simulink model "GScaleModelTrain_FuelCell"  (R2025b)
settings: Solver=ode23t  StartTime=0.0  StopTime=10  FixedStep=0.001  RelTol=1e-3
values from neighbouring files (symbols this model uses):
  eff = 0.85    [GScaleModelMatlab.m]
  G = 30    [GScaleModelMatlab.m]
  Ke = 0.01275    [GScaleModelMatlab.m]
  Kt = 0.01275    [GScaleModelMatlab.m]
  L = 0.001    [GScaleModelMatlab.m]
  num_motors = 2    [GScaleModelMatlab.m]
  num_wheels = 8    [GScaleModelMatlab.m]
  r = 0.017    [GScaleModelMatlab.m]
  Rm = 2.1    [GScaleModelMatlab.m]
  train_mass = mass_loco + (N * mass_wag)    (= 10.5)    [DavisResistance.m]    (also in GScaleModelMatlab.m)
  Vtrack = 20    [GScaleModelMatlab.m]
  x01 = 0    [GScaleModelMatlab.m]
  x02 = -0.5225    [GScaleModelMatlab.m]
  x03 = -1.1225    [GScaleModelMatlab.m]
  x04 = -1.7225    [GScaleModelMatlab.m]
libraries: fl_lib x12, nesl_utility x11, ee_lib x4
settings Model: Creator=2311591M  LastModifiedBy=Rahul
settings DebuggingCC: AlgebraicLoopMsg=none
settings SimscapeCC: SimscapeLogType=all

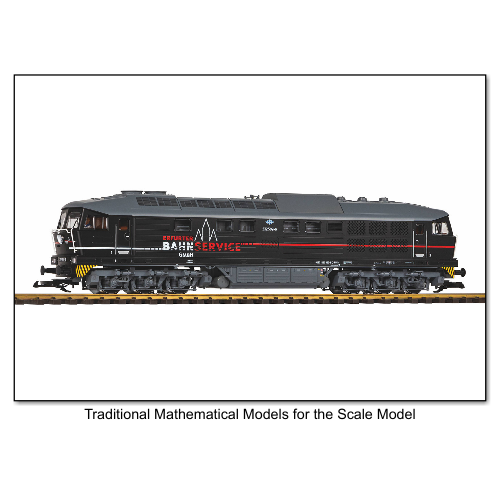
[thumbnail: Simulink's stored preview of the top-level diagram]
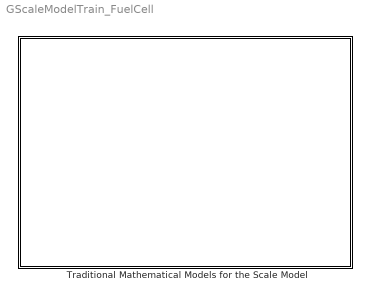
== system GScaleModelTrain_FuelCell ==
  Traditional Mathematical Models for the Scale Model : Subsystem
      mask Display: image('Luddy.jpg');

== system GScaleModelTrain_FuelCell/Traditional Mathematical Models for the Scale Model ==
  Combined Mass System : Subsystem
  Distributed Mass System : Subsystem
  Speed Visual : Scope  NumInputPorts=2
      settings: ActiveDisplayYMinimum=0.078796061919818139  ActiveDisplayYMaximum=1.1196711774107109  YLabel=Speed (m/s)  DataLoggingVariableName=ScopeData_3
  wires:
  Distributed Mass System/1(xd1) -> Speed Visual/2  "Distributed"
  Combined Mass System/1(xd) -> Speed Visual/1  "Combined"

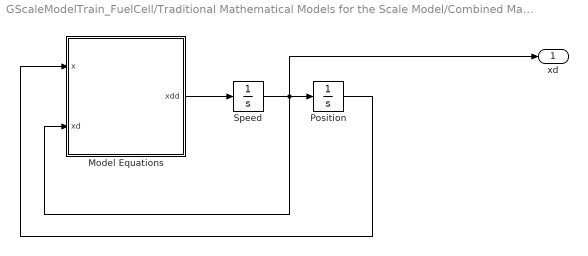
== system GScaleModelTrain_FuelCell/Traditional Mathematical Models for the Scale Model/Combined Mass System ==
  Model Equations : Subsystem
  Position : Integrator
  Speed : Integrator
  xd : Outport
  wires:
  Position/1 -> Model Equations/1(x)
  Model Equations/1(xdd) -> Speed/1
  Speed/1 -> xd/1, Model Equations/2(xd), Position/1

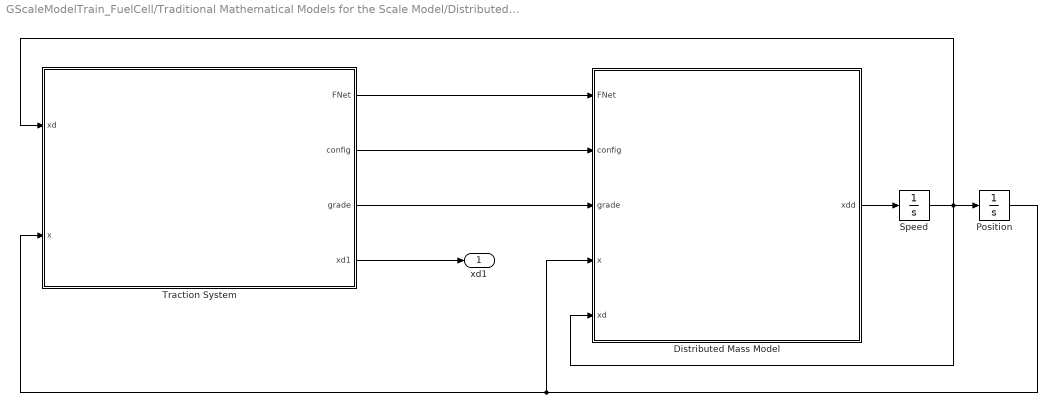
== system GScaleModelTrain_FuelCell/Traditional Mathematical Models for the Scale Model/Distributed Mass System ==
  Distributed Mass Model : MATLAB Function  TreatAsAtomicUnit=on
  Position : Integrator  InitialCondition=[x01; x02; x03; x04]
  Speed : Integrator
  Traction System : Subsystem
  xd1 : Outport
  wires:
  Traction System/4(xd1) -> xd1/1
  Traction System/3(grade) -> Distributed Mass Model/3(grade)
  Traction System/2(config) -> Distributed Mass Model/2(config)
  Traction System/1(FNet) -> Distributed Mass Model/1(FNet)
  Position/1 -> Distributed Mass Model/4(x), Traction System/2(x)
  Speed/1 -> Traction System/1(xd), Distributed Mass Model/5(xd), Position/1
  Distributed Mass Model/1(xdd) -> Speed/1

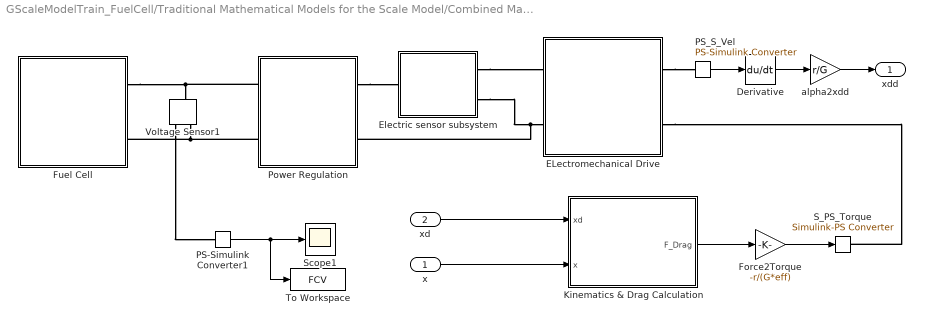
== system GScaleModelTrain_FuelCell/Traditional Mathematical Models for the Scale Model/Combined Mass System/Model Equations ==
  x : Inport
  xd : Inport  Port=2
  Derivative : Derivative
  ELectromechanical Drive : Subsystem
  Electric sensor subsystem : Subsystem
  Force2Torque : Gain  Gain=-r/(G*eff)
  Fuel Cell : Subsystem
  Kinematics & Drag Calculation : Subsystem
  PS-Simulink Converter1 : nesl_utility/PS-Simulink Converter  PhysicalDomain=network_engine_domain  SubClassName=ps_output  LeftPortType=input  RightPortType=output  PseudoPeriodic=off  Frequencies=[]  VectorFormat=inherit  Unit=inherit  AffineConversion=off
  PS_S_Vel : nesl_utility/PS-Simulink Converter  PhysicalDomain=network_engine_domain  SubClassName=ps_output  LeftPortType=input  RightPortType=output  PseudoPeriodic=off  Frequencies=[]  VectorFormat=inherit  Unit=inherit  AffineConversion=off
  Power Regulation : Subsystem
  S_PS_Torque : nesl_utility/Simulink-PS Converter  PhysicalDomain=network_engine_domain  SubClassName=ps_input  LeftPortType=input  RightPortType=output  PseudoPeriodic=off  Frequencies=[]  NoiseDistribution=none  NoiseParameters=[]  Unit=1  AffineConversion=off  FilteringAndDerivatives=filter  SimscapeFilterOrder=1  InputFilterTimeConstant=0.001  UdotUserProvided=0
  Scope1 : Scope
      settings: ActiveDisplayYMinimum=14.64179812710913  ActiveDisplayYMaximum=19.590394326626626
  To Workspace : ToWorkspace  VariableName=FCV  SaveFormat=Timeseries  SampleTime=-1
  Voltage Sensor1 : fl_lib/Electrical/Electrical Sensors/Voltage Sensor
  alpha2xdd : Gain  Gain=r/G
  xdd : Outport
  wires:
  Force2Torque/1 -> S_PS_Torque/1
  Derivative/1 -> alpha2xdd/1
  alpha2xdd/1 -> xdd/1
  PS_S_Vel/1 -> Derivative/1
  PS-Simulink Converter1/1 -> To Workspace/1, Scope1/1
  x/1 -> Kinematics & Drag Calculation/2(x)
  xd/1 -> Kinematics & Drag Calculation/1(xd)
  Kinematics & Drag Calculation/1(F_Drag) -> Force2Torque/1
  connections:
  Fuel Cell/RConn1 -- Power Regulation/LConn1 -- Voltage Sensor1/LConn1
  Voltage Sensor1/RConn1 -- PS-Simulink Converter1/LConn1
  Voltage Sensor1/RConn2 -- Fuel Cell/RConn2 -- Power Regulation/LConn2
  ELectromechanical Drive/RConn1 -- PS_S_Vel/LConn1
  ELectromechanical Drive/RConn2 -- S_PS_Torque/RConn1
  ELectromechanical Drive/LConn2 -- Electric sensor subsystem/RConn2 -- Power Regulation/RConn2
  Power Regulation/RConn1 -- Electric sensor subsystem/LConn1
  Electric sensor subsystem/RConn1 -- ELectromechanical Drive/LConn1

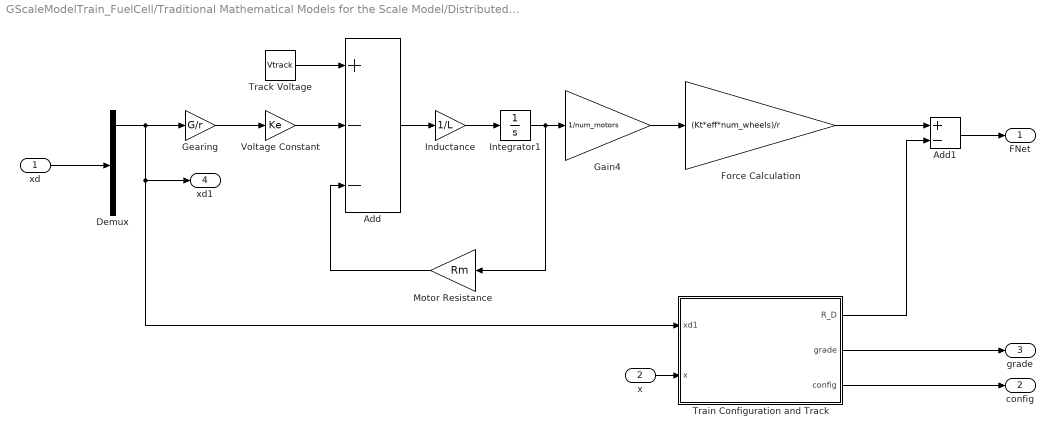
== system GScaleModelTrain_FuelCell/Traditional Mathematical Models for the Scale Model/Distributed Mass System/Traction System ==
  xd : Inport
  x : Inport  Port=2
  Add : Sum  Inputs=+--
  Add1 : Sum  Inputs=+-
  Demux : Demux
  Force Calculation : Gain  Gain=(Kt*eff*num_wheels)/r
  Gain4 : Gain  Gain=1/num_motors
  Gearing : Gain  Gain=G/r
  Inductance : Gain  Gain=1/L
  Integrator1 : Integrator
  Motor Resistance : Gain  Gain=Rm
  Track Voltage : Constant  Value=Vtrack
  Train Configuration and Track : Subsystem
  Voltage Constant : Gain  Gain=Ke
  FNet : Outport
  config : Outport  Port=2
  grade : Outport  Port=3
  xd1 : Outport  Port=4
  wires:
  Motor Resistance/1 -> Add/3
  Demux/1 -> Train Configuration and Track/1(xd1), xd1/1, Gearing/1
  Add/1 -> Inductance/1
  Inductance/1 -> Integrator1/1
  Voltage Constant/1 -> Add/2
  Gain4/1 -> Force Calculation/1
  Integrator1/1 -> Gain4/1, Motor Resistance/1
  Gearing/1 -> Voltage Constant/1
  Force Calculation/1 -> Add1/1
  xd/1 -> Demux/1
  Add1/1 -> FNet/1
  Track Voltage/1 -> Add/1
  x/1 -> Train Configuration and Track/2(x)
  Train Configuration and Track/1(R_D) -> Add1/2
  Train Configuration and Track/2(grade) -> grade/1
  Train Configuration and Track/3(config) -> config/1

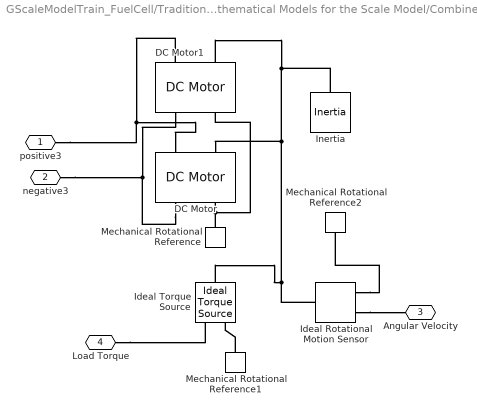
== system GScaleModelTrain_FuelCell/Traditional Mathematical Models for the Scale Model/Combined Mass System/Model Equations/ELectromechanical Drive ==
  DC Motor : ee_lib/Electromechanical/Brushed Motors/DC Motor  field_option=ee.enum.field_option.pm  Rf=100 Ohm  Lf=1 H  Laf=0.15 H  If0=0 A  parameterization=ee.enum.dcparam_option.circuit_param  Ra=Rm Ohm  La=L H  emf_or_torque=ee.enum.emf_or_torque.kv  Kv=Ke V/(rad/s)  Ki=0.01275 N*m/A  T_stall=0.24e-3 N*m  w_max=19100 rpm  w_rated=15000 rpm  P_rated=0.08 W  V_rated=1.5 V  lam_param=ee.enum.lam_param.damping  i_noload=0 A  V_i_noload=1.5 V  J=0.01 cm^2*g  lam=0 N*m*s/rad  speed0=0 rpm  alpha=3.93e-3 1/K  Tmeas=25 degC  thermal_mass=100 J/K  initial_temperature=25 degC
  DC Motor1 : ee_lib/Electromechanical/Brushed Motors/DC Motor  field_option=ee.enum.field_option.pm  Rf=100 Ohm  Lf=1 H  Laf=0.15 H  If0=0 A  parameterization=ee.enum.dcparam_option.circuit_param  Ra=Rm Ohm  La=L H  emf_or_torque=ee.enum.emf_or_torque.kv  Kv=Ke V/(rad/s)  Ki=0.01275 N*m/A  T_stall=0.24e-3 N*m  w_max=19100 rpm  w_rated=15000 rpm  P_rated=0.08 W  V_rated=1.5 V  lam_param=ee.enum.lam_param.damping  i_noload=0 A  V_i_noload=1.5 V  J=0.01 cm^2*g  lam=0 N*m*s/rad  speed0=0 rpm  alpha=3.93e-3 1/K  Tmeas=25 degC  thermal_mass=100 J/K  initial_temperature=25 degC
  Ideal Rotational Motion Sensor : fl_lib/Mechanical/Mechanical Sensors/Ideal Rotational Motion Sensor  reference=foundation.enum.MeasurementReference.difference  acceleration_port=false  velocity_port=true  position_port=false  wrap_angle=false  offset=0 rad
      settings: InternalSimscapePortConfiguration="{\"Bottom\":[],\"Left\":[{\"id\":\"R\",\"label\":\"R\",\"type\":\"foundation.mechanical.rotational.rotational\"}],\"Right\":[{\"id\":\"C\",\"label\":\"C\",\"type\":\"foundation.mechanical.rotational.rotational\"},{\"id\":\"W\",\"label\":\"W\",\"type\":\"output\"}],\"Top\":[]}"
  Ideal Torque Source : fl_lib/Mechanical/Mechanical Sources/Ideal Torque Source
  "Inertia " : fl_lib/Mechanical/Rotational Elements/Inertia  inertia=(train_mass * ( (r/G)^2) ) kg*m^2  num_ports=foundation.enum.numPorts2.one  w_specify=off  w_priority=High  w=0 rad/s  w_nominal_specify=off  w_nominal_value=1  w_nominal_unit=rad/s  t_specify=off  t_priority=None  t=0 N*m  t_nominal_specify=off  t_nominal_value=1  t_nominal_unit=N*m
  Mechanical Rotational Reference : fl_lib/Mechanical/Rotational Elements/Mechanical Rotational Reference
  Mechanical Rotational Reference1 : fl_lib/Mechanical/Rotational Elements/Mechanical Rotational Reference
  Mechanical Rotational Reference2 : fl_lib/Mechanical/Rotational Elements/Mechanical Rotational Reference
  positive3 : PMIOPort  Side=Left
  negative3 : PMIOPort  Port=2  Side=Left
  Angular Velocity : PMIOPort  Port=3  Side=Right
  Load Torque : PMIOPort  Port=4  Side=Right
  connections:
  DC Motor/RConn1 -- negative3/RConn1 -- DC Motor1/RConn1
  Mechanical Rotational Reference/LConn1 -- DC Motor1/RConn2 -- DC Motor/RConn2
  DC Motor1/LConn2 -- Ideal Torque Source/LConn1 -- Ideal Rotational Motion Sensor/LConn1 -- DC Motor/LConn2 -- "Inertia "/LConn1
  Ideal Rotational Motion Sensor/RConn2 -- Angular Velocity/RConn1
  Ideal Rotational Motion Sensor/RConn1 -- Mechanical Rotational Reference2/LConn1
  DC Motor1/LConn1 -- positive3/RConn1 -- DC Motor/LConn1
  Load Torque/RConn1 -- Ideal Torque Source/RConn1
  Mechanical Rotational Reference1/LConn1 -- Ideal Torque Source/RConn2

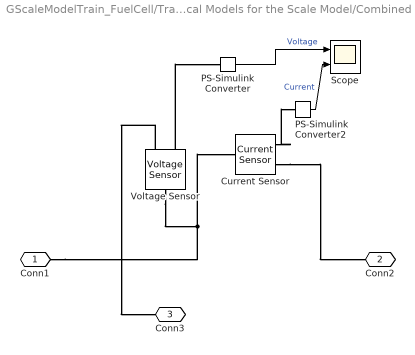
== system GScaleModelTrain_FuelCell/Traditional Mathematical Models for the Scale Model/Combined Mass System/Model Equations/Electric sensor subsystem ==
  Current Sensor : fl_lib/Electrical/Electrical Sensors/Current Sensor
  PS-Simulink Converter : nesl_utility/PS-Simulink Converter  PhysicalDomain=network_engine_domain  SubClassName=ps_output  LeftPortType=input  RightPortType=output  PseudoPeriodic=off  Frequencies=[]  VectorFormat=inherit  Unit=inherit  AffineConversion=off
  PS-Simulink Converter2 : nesl_utility/PS-Simulink Converter  PhysicalDomain=network_engine_domain  SubClassName=ps_output  LeftPortType=input  RightPortType=output  PseudoPeriodic=off  Frequencies=[]  VectorFormat=inherit  Unit=inherit  AffineConversion=off
  Scope : Scope  NumInputPorts=2
      settings: ActiveDisplayYMinimum=-1.7500040602157951  ActiveDisplayYMaximum=15.75003654394216  DataLoggingVariableName=ScopeData_1
  Voltage Sensor : fl_lib/Electrical/Electrical Sensors/Voltage Sensor
  Conn1 : PMIOPort  Side=Left
  Conn2 : PMIOPort  Port=2  Side=Right
  Conn3 : PMIOPort  Port=3  Side=Right
  wires:
  PS-Simulink Converter2/1 -> Scope/2  "Current"
  PS-Simulink Converter/1 -> Scope/1  "Voltage"
  connections:
  Current Sensor/RConn1 -- PS-Simulink Converter2/LConn1
  Voltage Sensor/RConn2 -- Conn3/RConn1
  Voltage Sensor/LConn1 -- Conn1/RConn1 -- Current Sensor/LConn1
  Voltage Sensor/RConn1 -- PS-Simulink Converter/LConn1
  Current Sensor/RConn2 -- Conn2/RConn1

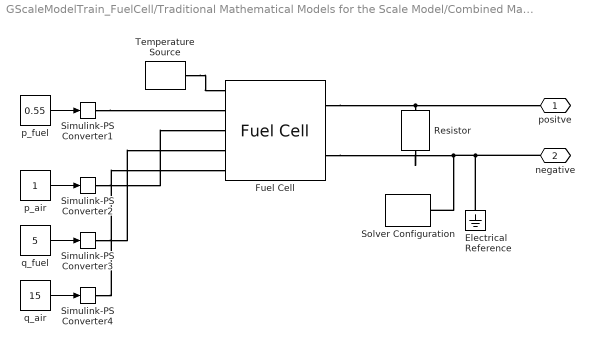
== system GScaleModelTrain_FuelCell/Traditional Mathematical Models for the Scale Model/Combined Mass System/Model Equations/Fuel Cell ==
  Electrical Reference : fl_lib/Electrical/Electrical Elements/Electrical Reference
  Fuel Cell : ee_lib/Sources/Fuel Cell  model_fidelity=ee.enum.fuelcell.fidelity.detailed  Eoc=19.1 V  A=0.125 V  ri=0.2 Ohm  i0=0.1 A  i_lim=10 A  N_cell=20  number_unit=1  pH2_nom=0.55 bar  pO2_nom=1 bar  xH2=99  xO2=21  xW=1  dyn=ee.enum.include.no  Rd=0.005 Ohm  tau=10 s  Tnom=293.15 K  thermal_mass=30000 J/K  iFC_specify=off  iFC_priority=None  iFC=1 A  iFC_nominal_specify=off  iFC_nominal_value=1  iFC_nominal_unit=A  vFC_specify=off  vFC_priority=None  vFC=0 V  vFC_nominal_specify=off  vFC_nominal_value=1  vFC_nominal_unit=V  temperature_specify=off  temperature_priority=High  temperature=293 K  temperature_nominal_specify=off  temperature_nominal_value=1  temperature_nominal_unit=K
      settings: InternalSimscapePortConfiguration="{\"Bottom\":[],\"Left\":[{\"id\":\"H\",\"label\":\"H\",\"type\":\"foundation.thermal.thermal\"},{\"id\":\"pfuel\",\"label\":\"pfuel\",\"type\":\"input\"},{\"id\":\"pair\",\"label\":\"pair\",\"type\":\"input\"},{\"id\":\"qfuel\",\"label\":\"qfuel\",\"type\":\"input\"},{\"id\":\"qair\",\"label\":\"qair\",\"type\":\"input\"}],\"Right\":[{\"id\":\"p\",\"label\":\"+\",\"type\":\"foundation.electrical.electrical\"},{\"id\":\"n\",\"label\":\"-\",\"type\":\"foundation.electrical.electrical\"}],\"Top\":[]}"
  Resistor : fl_lib/Electrical/Electrical Elements/Resistor  R=1000 Ohm  i_specify=off  i_priority=None  i=0 A  i_nominal_specify=off  i_nominal_value=1  i_nominal_unit=A  v_specify=off  v_priority=None  v=0 V  v_nominal_specify=off  v_nominal_value=1  v_nominal_unit=V
  Simulink-PS Converter1 : nesl_utility/Simulink-PS Converter  PhysicalDomain=network_engine_domain  SubClassName=ps_input  LeftPortType=input  RightPortType=output  PseudoPeriodic=off  Frequencies=[]  NoiseDistribution=none  NoiseParameters=[]  Unit=bar  AffineConversion=off  FilteringAndDerivatives=provide  SimscapeFilterOrder=1  InputFilterTimeConstant=0.001  UdotUserProvided=0
  Simulink-PS Converter2 : nesl_utility/Simulink-PS Converter  PhysicalDomain=network_engine_domain  SubClassName=ps_input  LeftPortType=input  RightPortType=output  PseudoPeriodic=off  Frequencies=[]  NoiseDistribution=none  NoiseParameters=[]  Unit=bar  AffineConversion=off  FilteringAndDerivatives=provide  SimscapeFilterOrder=1  InputFilterTimeConstant=0.001  UdotUserProvided=0
  Simulink-PS Converter3 : nesl_utility/Simulink-PS Converter  PhysicalDomain=network_engine_domain  SubClassName=ps_input  LeftPortType=input  RightPortType=output  PseudoPeriodic=off  Frequencies=[]  NoiseDistribution=none  NoiseParameters=[]  Unit=lpm  AffineConversion=off  FilteringAndDerivatives=provide  SimscapeFilterOrder=1  InputFilterTimeConstant=0.001  UdotUserProvided=0
  Simulink-PS Converter4 : nesl_utility/Simulink-PS Converter  PhysicalDomain=network_engine_domain  SubClassName=ps_input  LeftPortType=input  RightPortType=output  PseudoPeriodic=off  Frequencies=[]  NoiseDistribution=none  NoiseParameters=[]  Unit=lpm  AffineConversion=off  FilteringAndDerivatives=provide  SimscapeFilterOrder=1  InputFilterTimeConstant=0.001  UdotUserProvided=0
  Solver Configuration : nesl_utility/Solver Configuration  PhysicalDomain=network_engine_domain  SubClassName=solver  LeftPortType=input  RightPortType=generic  Tones=[]  Harmonics=[]  SimulateNoise=off  Profile=off  UseLocalSampling=off  EnableSwitchedLinearOptims=on  FrequencyDomain=off  UseCCode=off  RelTol=0.001  AbsTol=0.001  MinStep=1e-09  ToWorkspace=off  RevertToSquareIcSolve=off  NumHomotopyIterations=100  PhasorMode=off  PhasorModeNumHarmonics=1  ConsistencySolver=NEWTON_XTOL_AFTER_FTOL  IndexReductionMethod=DerivativeReplacement  DoDC=off  ResidualTolerance=1e-09  ConsistencyTolSource=GLOBAL  ConsistencyAbsTol=0.001  ConsistencyRelTol=0.001  ConsistencyTolFactor=0.001  UseLocalSolver=off  LocalSolverChoice=NE_BACKWARD_EULER_ADVANCER  ResolveIndetEquations=on  FunctionEvalNumThread=1  LocalSolverSampleTime=0.001  DoFixedCost=off  MaxNonlinIter=3  MaxModeIter=2  ComputeImpulses=off  ImpulseIterations=2  LinearAlgebra=auto  LinearAlgebraNumThread=0  EquationFormulation=NE_TIME_EF  DelaysMemoryBudget=1024  AutomaticFiltering=on  FilteringTimeConstant=0.001  PartitionStorageMethod=AS_NEEDED  PartitionMemoryBudget=1024  PartitionMethod=ROBUST  MultibodyUseLocalSolver=off  MultibodyLocalSolverChoice=ODE1  MultibodyLocalSolverSampleTime=0.001
  Temperature Source : fl_lib/Thermal/Thermal Sources/Temperature Source  temperature=293.15 K
  p_air : Constant
  p_fuel : Constant  Value=0.55
  q_air : Constant  Value=15
  q_fuel : Constant  Value=5
  positve : PMIOPort  Side=Right
  negative : PMIOPort  Port=2  Side=Right
  wires:
  p_fuel/1 -> Simulink-PS Converter1/1
  q_air/1 -> Simulink-PS Converter4/1
  q_fuel/1 -> Simulink-PS Converter3/1
  p_air/1 -> Simulink-PS Converter2/1
  connections:
  Electrical Reference/LConn1 -- negative/RConn1 -- Solver Configuration/RConn1 -- Resistor/RConn1 -- Fuel Cell/RConn2
  Temperature Source/LConn1 -- Fuel Cell/LConn1
  Simulink-PS Converter1/RConn1 -- Fuel Cell/LConn2
  Fuel Cell/RConn1 -- Resistor/LConn1 -- positve/RConn1
  Simulink-PS Converter4/RConn1 -- Fuel Cell/LConn5
  Simulink-PS Converter2/RConn1 -- Fuel Cell/LConn3
  Simulink-PS Converter3/RConn1 -- Fuel Cell/LConn4

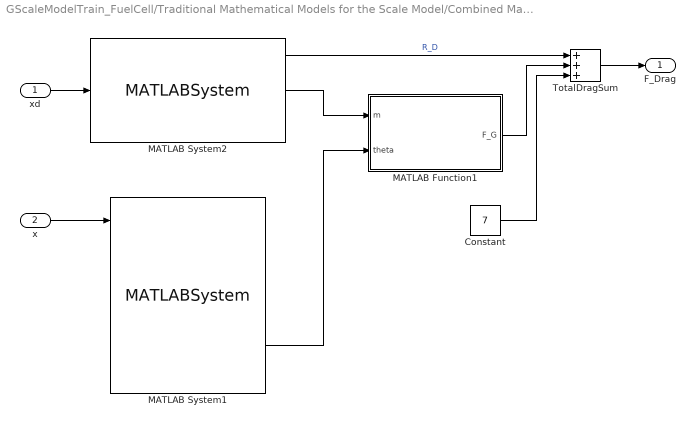
== system GScaleModelTrain_FuelCell/Traditional Mathematical Models for the Scale Model/Combined Mass System/Model Equations/Kinematics & Drag Calculation ==
  xd : Inport
  x : Inport  Port=2
  Constant : Constant  Value=7
  MATLAB Function1 : MATLAB Function  TreatAsAtomicUnit=on
  MATLAB System1 : MATLABSystem  System=Track  SimulateUsing=Code generation
      mask Type: Track
  MATLAB System2 : MATLABSystem  System=DavisResistance  SimulateUsing=Code generation
      mask Type: DavisResistance
  TotalDragSum : Sum  Inputs=+++
  F_Drag : Outport
  wires:
  MATLAB System2/2 -> MATLAB Function1/1(m)
  x/1 -> MATLAB System1/1
  MATLAB System1/2 -> MATLAB Function1/2(theta)
  xd/1 -> MATLAB System2/1
  Constant/1 -> TotalDragSum/3
  MATLAB Function1/1(F_G) -> TotalDragSum/2
  TotalDragSum/1 -> F_Drag/1
  MATLAB System2/1 -> TotalDragSum/1  "R_D"

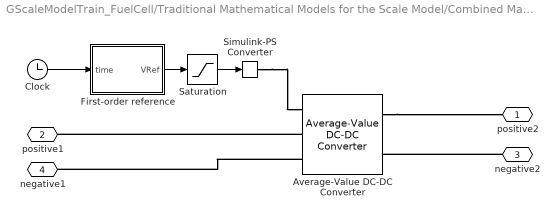
== system GScaleModelTrain_FuelCell/Traditional Mathematical Models for the Scale Model/Combined Mass System/Model Equations/Power Regulation ==
  Average-Value DC-DC Converter : ee_lib/Semiconductors & Converters/Converters/Average-Value DC-DC Converter  implementation_option=ee.enum.converters.implementation.behavioral  converter_type=ee.enum.converters.dcdctype.buck  control_option=ee.enum.converters.controlinput.voltage  efficiency_option=ee.enum.converters.efficiency.constant  efficiency_fixed=100  i_vec=[0, 2, 5] A  efficiency_vec=[90, 95, 98]  Lf=1e-6 H  Rl=1e-3 Ohm  Cf=1e-7 F  Rc=1e-3 Ohm  iL_specify=off  iL_priority=High  iL=0 A  iL_nominal_specify=off  iL_nominal_value=1  iL_nominal_unit=A  vc_specify=on  vc_priority=High  vc=0 V  vc_nominal_specify=on  vc_nominal_value=0  vc_nominal_unit=V
      settings: InternalSimscapePortConfiguration="{\"Bottom\":[],\"Left\":[{\"id\":\"Vref\",\"label\":\"Vref\",\"type\":\"input\"},{\"id\":\"p1\",\"label\":\"1+\",\"type\":\"foundation.electrical.electrical\"},{\"id\":\"n1\",\"label\":\"1-\",\"type\":\"foundation.electrical.electrical\"}],\"Right\":[{\"id\":\"p2\",\"label\":\"2+\",\"type\":\"foundation.electrical.electrical\"},{\"id\":\"n2\",\"label\":\"2-\",\"type\":\"foundation.electrical.electrical\"}],\"Top\":[]}"
  Clock : Clock
  First-order reference : MATLAB Function  TreatAsAtomicUnit=on
  Saturation : Saturate  UpperLimit=14  LowerLimit=0.1
  Simulink-PS Converter : nesl_utility/Simulink-PS Converter  PhysicalDomain=network_engine_domain  SubClassName=ps_input  LeftPortType=input  RightPortType=output  PseudoPeriodic=off  Frequencies=[]  NoiseDistribution=none  NoiseParameters=[]  Unit=V  AffineConversion=off  FilteringAndDerivatives=filter  SimscapeFilterOrder=1  InputFilterTimeConstant=0.001  UdotUserProvided=0
  positive2 : PMIOPort  Side=Right
  positive1 : PMIOPort  Port=2  Side=Left
  negative2 : PMIOPort  Port=3  Side=Right
  negative1 : PMIOPort  Port=4  Side=Left
  wires:
  Saturation/1 -> Simulink-PS Converter/1
  First-order reference/1(VRef) -> Saturation/1
  Clock/1 -> First-order reference/1(time)
  connections:
  Average-Value DC-DC Converter/RConn1 -- positive2/RConn1
  Simulink-PS Converter/RConn1 -- Average-Value DC-DC Converter/LConn1
  negative2/RConn1 -- Average-Value DC-DC Converter/RConn2
  Average-Value DC-DC Converter/LConn3 -- negative1/RConn1
  Average-Value DC-DC Converter/LConn2 -- positive1/RConn1

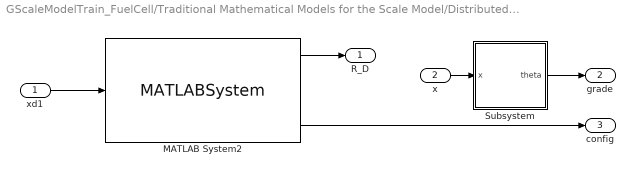
== system GScaleModelTrain_FuelCell/Traditional Mathematical Models for the Scale Model/Distributed Mass System/Traction System/Train Configuration and Track ==
  xd1 : Inport
  x : Inport  Port=2
  MATLAB System2 : MATLABSystem  System=DavisResistance  SimulateUsing=Code generation
      mask Type: DavisResistance
  Subsystem : Subsystem
  R_D : Outport
  grade : Outport  Port=2
  config : Outport  Port=3
  wires:
  Subsystem/1(theta) -> grade/1
  MATLAB System2/3 -> config/1
  x/1 -> Subsystem/1(x)
  MATLAB System2/1 -> R_D/1
  xd1/1 -> MATLAB System2/1

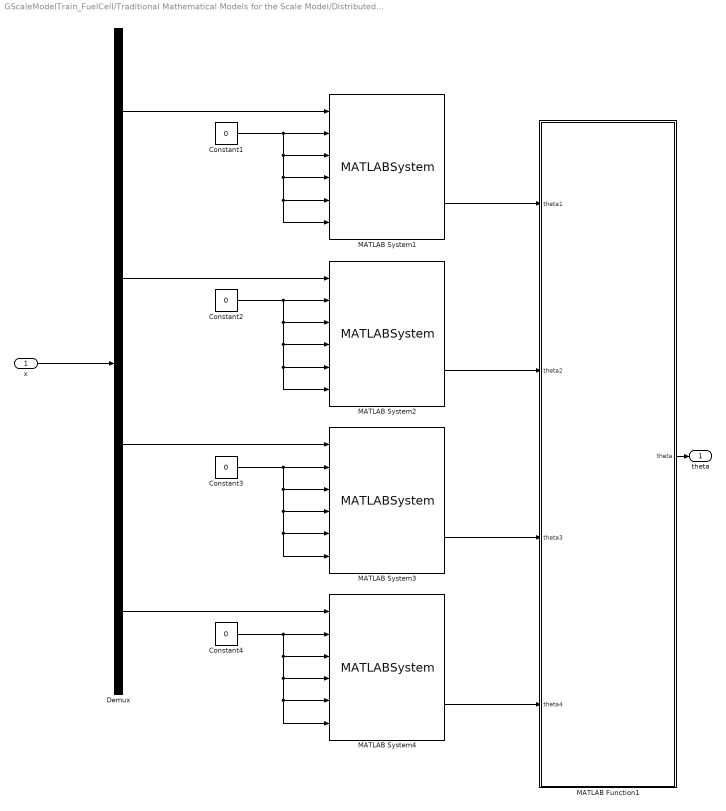
== system GScaleModelTrain_FuelCell/Traditional Mathematical Models for the Scale Model/Distributed Mass System/Traction System/Train Configuration and Track/Subsystem ==
  x : Inport
  Constant{1..4} (4 alike) : Constant  Value=0
  Demux : Demux
  MATLAB Function1 : MATLAB Function  TreatAsAtomicUnit=on
  MATLAB System{1..4} (4 alike) : MATLABSystem  System=Track  SimulateUsing=Code generation
      mask Type: Track
  theta : Outport
  wires:
  Constant1/1 -> MATLAB System1/6, MATLAB System1/5, MATLAB System1/4, MATLAB System1/3, MATLAB System1/2
  MATLAB Function1/1(theta) -> theta/1
  Constant2/1 -> MATLAB System2/6, MATLAB System2/5, MATLAB System2/4, MATLAB System2/3, MATLAB System2/2
  Constant3/1 -> MATLAB System3/6, MATLAB System3/5, MATLAB System3/4, MATLAB System3/3, MATLAB System3/2
  Constant4/1 -> MATLAB System4/6, MATLAB System4/5, MATLAB System4/4, MATLAB System4/3, MATLAB System4/2
  x/1 -> Demux/1
  Demux/1 -> MATLAB System1/1
  Demux/2 -> MATLAB System2/1
  Demux/3 -> MATLAB System3/1
  Demux/4 -> MATLAB System4/1
  MATLAB System4/2 -> MATLAB Function1/4(theta4)
  MATLAB System3/2 -> MATLAB Function1/3(theta3)
  MATLAB System2/2 -> MATLAB Function1/2(theta2)
  MATLAB System1/2 -> MATLAB Function1/1(theta1)

== matlab function GScaleModelTrain_FuelCell/Traditional Mathematical Models for the Scale Model/Combined Mass System/Model Equations/Power Regulation/First-order reference ==
  data: time input; VRef output
function VRef = fcn(time)
Vlim = 14;
sigma =2.75;

VRef = Vlim * (1 - exp(-sigma * time));

end

== matlab function GScaleModelTrain_FuelCell/Traditional Mathematical Models for the Scale Model/Distributed Mass System/Distributed Mass Model ==
  data: FNet input; config input; grade input; x input; xd input; xdd output
function xdd = DistributedMassModel(FNet, config, grade, x, xd)

% Mass
m = [10.5; 8; 8; 8];

% Coupler
k = 6500;    % spring N/m
c = 65;     % damper N/(m/s)

d12 = 0.5225;
d23 = 0.6;
d34 = 0.6;

Nmax = 4;
xdd = zeros(Nmax,1);

F_c = zeros(Nmax-1,1);  % coupler forces between units

% Calculate coupler forces for active cars
if config >= 2
    F_c(1) = k*((x(1)-x(2))-d12) + c*(xd(1)-xd(2));
end
if config >= 3
    F_c(2) = k*((x(2)-x(3))-d23) + c*(xd(2)-xd(3));
end
if config >= 4
    F_c(3) = k*((x(3)-x(4))-d34) + c*(xd(3)-xd(4));
end

% Acceleration Equations
for i = 1:Nmax
    
    % Skip inactive vehicles
    if i > config
        xdd(i) = 0;
        continue
    end
    
    % --- RESISTANCE ---
    g = 9.81;
    F_grade = m(i)*g*sind(grade(i));
    F_res = F_grade;
    
    % --- TRACTION ---
    if i == 1
        F_trac = FNet;
    else
        F_trac = 0;
    end
    
    % --- COUPLER INTERACTIONS ---
    F_prev = 0;  % force from car ahead
    F_next = 0;  % force from car behind
    
    if i > 1 && (i-1) <= config-1
        F_prev = F_c(i-1);  % force pulling/pushing from previous car
    end
    if i < config
        F_next = F_c(i);    % force pushing/pulling from next car
    end
    
    % Net Acceleration
    % Forces on car: traction + couplers - resistance
    xdd(i) = (F_trac - F_res + F_prev - F_next) / m(i);
end
end

== matlab function GScaleModelTrain_FuelCell/Traditional Mathematical Models for the Scale Model/Distributed Mass System/Traction System/Train Configuration and Track/Subsystem/MATLAB Function1 ==
  data: theta1 input; theta output; theta2 input; theta3 input; theta4 input
function theta = GradientForce(theta1,theta2,theta3,theta4)

theta = [theta1; theta2; theta3; theta4];  % radians

end

== matlab function GScaleModelTrain_FuelCell/Traditional Mathematical Models for the Scale Model/Combined Mass System/Model Equations/Kinematics & Drag Calculation/MATLAB Function1 ==
  data: m input; theta input; F_G output
function F_G = GradientForce(m,theta)

g = 9.81;

F_G = m * g * sind(theta);
